simulink model "lineFollow_onoff_soln"  (R2018a)
settings: Solver=FixedStepDiscrete  StartTime=0.0  StopTime=360  FixedStep=0.01  RelTol=1e-3
PreLoadFcn:
  | robotParameters;
  | load exampleLineFollowingMap.mat
undefined symbols (not defined in the file): motorIp, motorSp
libraries: mobileRoboticsTrainingLib x5
settings Model: Creator=sseshadr  LastModifiedBy=whaj47
settings CodeAppCC: StateflowObjectComments=on

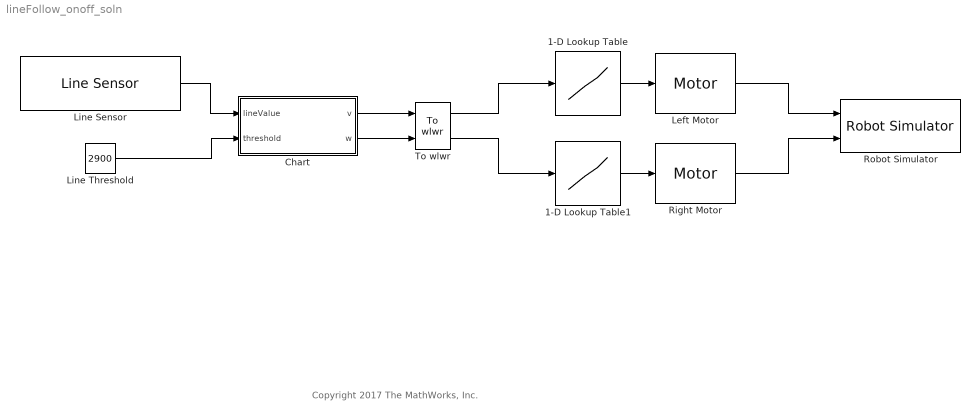
== system lineFollow_onoff_soln ==
  note: Copyright 2017 The MathWorks, Inc.
  1-D Lookup Table : Lookup_n-D  NumberOfTableDimensions=1  BreakpointsForDimension1=motorSp  Table=motorIp  ExtrapMethod=Clip  InternalRulePriority=Speed  RndMeth=Simplest  InputSameDT=on
  1-D Lookup Table1 : Lookup_n-D  NumberOfTableDimensions=1  BreakpointsForDimension1=motorSp  Table=motorIp  ExtrapMethod=Clip  InternalRulePriority=Speed  RndMeth=Simplest  InputSameDT=on
  Chart : Stateflow chart  TreatAsAtomicUnit=on
  Left Motor : mobileRoboticsTrainingLib/Motor  motorPlant=wheelMotorModel  sensorType=Speed
      settings: SourceProductName=Mobile Robotics Training Library
  Line Sensor : mobileRoboticsTrainingLib/Line Sensor  mapVariable=mapForSim  envVal=2850  lineVal=2950  sensOff=[0.01 0]
      settings: SourceProductName=Mobile Robotics Training Library
  Line Threshold : Constant  Value=2900
  Right Motor : mobileRoboticsTrainingLib/Motor  motorPlant=wheelMotorModel  sensorType=Speed
      settings: SourceProductName=Mobile Robotics Training Library
  Robot Simulator : mobileRoboticsTrainingLib/Robot Simulator  Priority=99  mapVar=mapForSim  startX=0.62198  startY=1.3096  startTheta=0  axleLength=axleLength  wheelR=wheelR
  To wlwr : mobileRoboticsTrainingLib/To wlwr  axleLength=axleLength  wheelR=wheelR
  wires:
  Left Motor/1 -> Robot Simulator/1
  1-D Lookup Table1/1 -> Right Motor/1
  1-D Lookup Table/1 -> Left Motor/1
  Right Motor/1 -> Robot Simulator/2
  To wlwr/1 -> 1-D Lookup Table/1
  To wlwr/2 -> 1-D Lookup Table1/1
  Chart/1(v) -> To wlwr/1
  Chart/2(w) -> To wlwr/2
  Line Sensor/1 -> Chart/1(lineValue)
  Line Threshold/1 -> Chart/2(threshold)

== stateflow chart lineFollow_onoff_soln/Chart ==
  state GoLeft
    entry:
    v = 0.05;
    w = 1;
  state GoRight
    entry:
    v = 0.05;
    w = -1;
  (default) -> GoLeft
  GoLeft -> GoRight : [lineValue < threshold]
  GoRight -> GoLeft : [lineValue >= threshold]
  data: v output; w output; lineValue input; threshold input
